simulink model "RADTRANS002"  (R2020b)
settings: Solver=VariableStepAuto  StartTime=0.0  StopTime=10.0  RelTol=1e-3
undefined symbols (not defined in the file): Line_110_C, Line_110_L, Line_110_R, Line_220_C, Line_220_L, Line_220_R, Line_35_C, Line_35_L, Line_35_R, Line_6_L, Line_6_R, Sys_f_Hz, Sys_V_net_kV, Tr_110_35_L_pu, Tr_110_35_R_pu, Tr_110_35_Sn_VA, Tr_110_35_V_HV_kV, Tr_110_35_V_LV_kV, Tr_110_6_L_pu, Tr_110_6_R_pu, Tr_110_6_Sn_VA, Tr_110_6_V_HV_kV, Tr_110_6_V_LV_kV, Tr_220_110_L_pu, Tr_220_110_R_pu, Tr_220_110_Sn_VA, Tr_220_110_V_HV_kV, Tr_220_110_V_LV_kV, Tr_35_04_L_pu, Tr_35_04_R_pu, Tr_35_04_Sn_VA, Tr_35_04_V_HV_kV, Tr_35_04_V_LV_kV, Tr_6_04_L_pu, Tr_6_04_R_pu, Tr_6_04_Sn_VA, Tr_6_04_V_HV_kV, Tr_6_04_V_LV_kV, Ts_powergui
libraries: dspstat3 x288, powerlib x202, powerlib_meascontrol x72
(part 6 of 7)

== system RADTRANS002/M_OUT_Город_4_4 ==
  Iptg_48 : Display
      settings: Format=bank
  PQptg_48 : Scope  NumInputPorts=2
  "Power0 (3ph, Instantaneous)" : powerlib_meascontrol/Measurements/Power (3ph, Instantaneous)
  Pptg_48 : Display
      settings: Format=bank
  Qptg_48 : Display
      settings: Format=bank
  RMS3 : dspstat3/RMS  run=off  directionMode=Each column  dimension=1  InputProcessing=Columns as channels (frame based)  reset_popup=None
  RMS4 : dspstat3/RMS  run=off  directionMode=Each column  dimension=1  InputProcessing=Columns as channels (frame based)  reset_popup=None
  RMS48 : dspstat3/RMS  run=off  directionMode=Each column  dimension=1  InputProcessing=Columns as channels (frame based)  reset_popup=None
  RMSpt_48 : dspstat3/RMS  run=off  directionMode=Each column  dimension=1  InputProcessing=Columns as channels (frame based)  reset_popup=None
  Real-Ima to Complex : RealImagToComplex
  S : Abs
  SSptg_48 : Scope
  Sptg_48 : Display
      settings: Format=bank
  Three-Phase V-I Measurementpt_48 : powerlib/Measurements/Three-Phase V-I Measurement  VoltageMeasurement=phase-to-ground  SetLabelV=off  LabelV=Vabc  Vpu=off  VpuLL=off  CurrentMeasurement=yes  SetLabelI=off  LabelI=Iabc  Ipu=off  Pbase=100e6  Vbase=500e3  OutputType=Complex  PhasorSimulation=off  PSBequivalent=0
  UIptg_48 : Scope  NumInputPorts=2
  Uptg_48 : Display
      settings: Format=bank
  a : PMIOPort  Side=Right
  b : PMIOPort  Port=2  Side=Right
  c : PMIOPort  Port=3  Side=Right
  A : PMIOPort  Port=4  Side=Left
  B : PMIOPort  Port=5  Side=Left
  C : PMIOPort  Port=6  Side=Left
  tag scope: I_ptg_48=global, P_ptg_48=global, Q_ptg_48=global, S_ptg_48=global, U_ptg_48=global
  wires:
  S/1 -> [S_ptg_48]
  Real-Ima to Complex/1 -> S/1
  [S_ptg_48] -> Sptg_48/1
  [S_ptg_48] -> SSptg_48/1
  [P_ptg_48] -> RMSpt_48/1
  RMSpt_48/1 -> Pptg_48/1
  RMS48/1 -> Qptg_48/1
  [U_ptg_48] -> RMS3/1
  RMS3/1 -> Uptg_48/1
  [P_ptg_48] -> Real-Ima to Complex/1
  [Q_ptg_48] -> RMS48/1
  [I_ptg_48] -> RMS4/1
  RMS4/1 -> Iptg_48/1
  [U_ptg_48] -> UIptg_48/1  "U"
  [P_ptg_48] -> PQptg_48/1  "P"
  [I_ptg_48] -> UIptg_48/2  "I"
  Three-Phase V-I Measurementpt_48/1 -> [U_ptg_48]
  [Q_ptg_48] -> Real-Ima to Complex/2
  Three-Phase V-I Measurementpt_48/2 -> [I_ptg_48]
  [U_ptg_48] -> "Power0 (3ph, Instantaneous)"/1
  [I_ptg_48] -> "Power0 (3ph, Instantaneous)"/2
  "Power0 (3ph, Instantaneous)"/2 -> [Q_ptg_48]
  "Power0 (3ph, Instantaneous)"/1 -> [P_ptg_48]
  [Q_ptg_48] -> PQptg_48/2  "Q"
  connections:
  Three-Phase V-I Measurementpt_48/LConn1 -- A/RConn1
  Three-Phase V-I Measurementpt_48/RConn1 -- a/RConn1
  Three-Phase V-I Measurementpt_48/LConn2 -- B/RConn1
  Three-Phase V-I Measurementpt_48/LConn3 -- C/RConn1
  Three-Phase V-I Measurementpt_48/RConn3 -- c/RConn1
  Three-Phase V-I Measurementpt_48/RConn2 -- b/RConn1

== system RADTRANS002/M_OUT_Город_5_1 ==
  Iptg_54 : Display
      settings: Format=bank
  PQptg_54 : Scope  NumInputPorts=2
  "Power0 (3ph, Instantaneous)" : powerlib_meascontrol/Measurements/Power (3ph, Instantaneous)
  Pptg_54 : Display
      settings: Format=bank
  Qptg_54 : Display
      settings: Format=bank
  RMS3 : dspstat3/RMS  run=off  directionMode=Each column  dimension=1  InputProcessing=Columns as channels (frame based)  reset_popup=None
  RMS4 : dspstat3/RMS  run=off  directionMode=Each column  dimension=1  InputProcessing=Columns as channels (frame based)  reset_popup=None
  RMS54 : dspstat3/RMS  run=off  directionMode=Each column  dimension=1  InputProcessing=Columns as channels (frame based)  reset_popup=None
  RMSpt_54 : dspstat3/RMS  run=off  directionMode=Each column  dimension=1  InputProcessing=Columns as channels (frame based)  reset_popup=None
  Real-Ima to Complex : RealImagToComplex
  S : Abs
  SSptg_54 : Scope
  Sptg_54 : Display
      settings: Format=bank
  Three-Phase V-I Measurementpt_54 : powerlib/Measurements/Three-Phase V-I Measurement  VoltageMeasurement=phase-to-ground  SetLabelV=off  LabelV=Vabc  Vpu=off  VpuLL=off  CurrentMeasurement=yes  SetLabelI=off  LabelI=Iabc  Ipu=off  Pbase=100e6  Vbase=500e3  OutputType=Complex  PhasorSimulation=off  PSBequivalent=0
  UIptg_54 : Scope  NumInputPorts=2
  Uptg_54 : Display
      settings: Format=bank
  a : PMIOPort  Side=Right
  b : PMIOPort  Port=2  Side=Right
  c : PMIOPort  Port=3  Side=Right
  A : PMIOPort  Port=4  Side=Left
  B : PMIOPort  Port=5  Side=Left
  C : PMIOPort  Port=6  Side=Left
  tag scope: I_ptg_54=global, P_ptg_54=global, Q_ptg_54=global, S_ptg_54=global, U_ptg_54=global
  wires:
  S/1 -> [S_ptg_54]
  Real-Ima to Complex/1 -> S/1
  [S_ptg_54] -> Sptg_54/1
  [S_ptg_54] -> SSptg_54/1
  [P_ptg_54] -> RMSpt_54/1
  RMSpt_54/1 -> Pptg_54/1
  RMS54/1 -> Qptg_54/1
  [U_ptg_54] -> RMS3/1
  RMS3/1 -> Uptg_54/1
  [P_ptg_54] -> Real-Ima to Complex/1
  [Q_ptg_54] -> RMS54/1
  [I_ptg_54] -> RMS4/1
  RMS4/1 -> Iptg_54/1
  [U_ptg_54] -> UIptg_54/1  "U"
  [P_ptg_54] -> PQptg_54/1  "P"
  [I_ptg_54] -> UIptg_54/2  "I"
  Three-Phase V-I Measurementpt_54/1 -> [U_ptg_54]
  [Q_ptg_54] -> Real-Ima to Complex/2
  Three-Phase V-I Measurementpt_54/2 -> [I_ptg_54]
  [U_ptg_54] -> "Power0 (3ph, Instantaneous)"/1
  [I_ptg_54] -> "Power0 (3ph, Instantaneous)"/2
  "Power0 (3ph, Instantaneous)"/2 -> [Q_ptg_54]
  "Power0 (3ph, Instantaneous)"/1 -> [P_ptg_54]
  [Q_ptg_54] -> PQptg_54/2  "Q"
  connections:
  Three-Phase V-I Measurementpt_54/LConn1 -- A/RConn1
  Three-Phase V-I Measurementpt_54/RConn1 -- a/RConn1
  Three-Phase V-I Measurementpt_54/LConn2 -- B/RConn1
  Three-Phase V-I Measurementpt_54/LConn3 -- C/RConn1
  Three-Phase V-I Measurementpt_54/RConn3 -- c/RConn1
  Three-Phase V-I Measurementpt_54/RConn2 -- b/RConn1

== system RADTRANS002/M_OUT_Город_5_2 ==
  Iptg_56 : Display
      settings: Format=bank
  PQptg_56 : Scope  NumInputPorts=2
  "Power0 (3ph, Instantaneous)" : powerlib_meascontrol/Measurements/Power (3ph, Instantaneous)
  Pptg_56 : Display
      settings: Format=bank
  Qptg_56 : Display
      settings: Format=bank
  RMS3 : dspstat3/RMS  run=off  directionMode=Each column  dimension=1  InputProcessing=Columns as channels (frame based)  reset_popup=None
  RMS4 : dspstat3/RMS  run=off  directionMode=Each column  dimension=1  InputProcessing=Columns as channels (frame based)  reset_popup=None
  RMS56 : dspstat3/RMS  run=off  directionMode=Each column  dimension=1  InputProcessing=Columns as channels (frame based)  reset_popup=None
  RMSpt_56 : dspstat3/RMS  run=off  directionMode=Each column  dimension=1  InputProcessing=Columns as channels (frame based)  reset_popup=None
  Real-Ima to Complex : RealImagToComplex
  S : Abs
  SSptg_56 : Scope
  Sptg_56 : Display
      settings: Format=bank
  Three-Phase V-I Measurementpt_56 : powerlib/Measurements/Three-Phase V-I Measurement  VoltageMeasurement=phase-to-ground  SetLabelV=off  LabelV=Vabc  Vpu=off  VpuLL=off  CurrentMeasurement=yes  SetLabelI=off  LabelI=Iabc  Ipu=off  Pbase=100e6  Vbase=500e3  OutputType=Complex  PhasorSimulation=off  PSBequivalent=0
  UIptg_56 : Scope  NumInputPorts=2
  Uptg_56 : Display
      settings: Format=bank
  a : PMIOPort  Side=Right
  b : PMIOPort  Port=2  Side=Right
  c : PMIOPort  Port=3  Side=Right
  A : PMIOPort  Port=4  Side=Left
  B : PMIOPort  Port=5  Side=Left
  C : PMIOPort  Port=6  Side=Left
  tag scope: I_ptg_56=global, P_ptg_56=global, Q_ptg_56=global, S_ptg_56=global, U_ptg_56=global
  wires:
  S/1 -> [S_ptg_56]
  Real-Ima to Complex/1 -> S/1
  [S_ptg_56] -> Sptg_56/1
  [S_ptg_56] -> SSptg_56/1
  [P_ptg_56] -> RMSpt_56/1
  RMSpt_56/1 -> Pptg_56/1
  RMS56/1 -> Qptg_56/1
  [U_ptg_56] -> RMS3/1
  RMS3/1 -> Uptg_56/1
  [P_ptg_56] -> Real-Ima to Complex/1
  [Q_ptg_56] -> RMS56/1
  [I_ptg_56] -> RMS4/1
  RMS4/1 -> Iptg_56/1
  [U_ptg_56] -> UIptg_56/1  "U"
  [P_ptg_56] -> PQptg_56/1  "P"
  [I_ptg_56] -> UIptg_56/2  "I"
  Three-Phase V-I Measurementpt_56/1 -> [U_ptg_56]
  [Q_ptg_56] -> Real-Ima to Complex/2
  Three-Phase V-I Measurementpt_56/2 -> [I_ptg_56]
  [U_ptg_56] -> "Power0 (3ph, Instantaneous)"/1
  [I_ptg_56] -> "Power0 (3ph, Instantaneous)"/2
  "Power0 (3ph, Instantaneous)"/2 -> [Q_ptg_56]
  "Power0 (3ph, Instantaneous)"/1 -> [P_ptg_56]
  [Q_ptg_56] -> PQptg_56/2  "Q"
  connections:
  Three-Phase V-I Measurementpt_56/LConn1 -- A/RConn1
  Three-Phase V-I Measurementpt_56/RConn1 -- a/RConn1
  Three-Phase V-I Measurementpt_56/LConn2 -- B/RConn1
  Three-Phase V-I Measurementpt_56/LConn3 -- C/RConn1
  Three-Phase V-I Measurementpt_56/RConn3 -- c/RConn1
  Three-Phase V-I Measurementpt_56/RConn2 -- b/RConn1

== system RADTRANS002/M_OUT_Город_5_3 ==
  Iptg_58 : Display
      settings: Format=bank
  PQptg_58 : Scope  NumInputPorts=2
  "Power0 (3ph, Instantaneous)" : powerlib_meascontrol/Measurements/Power (3ph, Instantaneous)
  Pptg_58 : Display
      settings: Format=bank
  Qptg_58 : Display
      settings: Format=bank
  RMS3 : dspstat3/RMS  run=off  directionMode=Each column  dimension=1  InputProcessing=Columns as channels (frame based)  reset_popup=None
  RMS4 : dspstat3/RMS  run=off  directionMode=Each column  dimension=1  InputProcessing=Columns as channels (frame based)  reset_popup=None
  RMS58 : dspstat3/RMS  run=off  directionMode=Each column  dimension=1  InputProcessing=Columns as channels (frame based)  reset_popup=None
  RMSpt_58 : dspstat3/RMS  run=off  directionMode=Each column  dimension=1  InputProcessing=Columns as channels (frame based)  reset_popup=None
  Real-Ima to Complex : RealImagToComplex
  S : Abs
  SSptg_58 : Scope
  Sptg_58 : Display
      settings: Format=bank
  Three-Phase V-I Measurementpt_58 : powerlib/Measurements/Three-Phase V-I Measurement  VoltageMeasurement=phase-to-ground  SetLabelV=off  LabelV=Vabc  Vpu=off  VpuLL=off  CurrentMeasurement=yes  SetLabelI=off  LabelI=Iabc  Ipu=off  Pbase=100e6  Vbase=500e3  OutputType=Complex  PhasorSimulation=off  PSBequivalent=0
  UIptg_58 : Scope  NumInputPorts=2
  Uptg_58 : Display
      settings: Format=bank
  a : PMIOPort  Side=Right
  b : PMIOPort  Port=2  Side=Right
  c : PMIOPort  Port=3  Side=Right
  A : PMIOPort  Port=4  Side=Left
  B : PMIOPort  Port=5  Side=Left
  C : PMIOPort  Port=6  Side=Left
  tag scope: I_ptg_58=global, P_ptg_58=global, Q_ptg_58=global, S_ptg_58=global, U_ptg_58=global
  wires:
  S/1 -> [S_ptg_58]
  Real-Ima to Complex/1 -> S/1
  [S_ptg_58] -> Sptg_58/1
  [S_ptg_58] -> SSptg_58/1
  [P_ptg_58] -> RMSpt_58/1
  RMSpt_58/1 -> Pptg_58/1
  RMS58/1 -> Qptg_58/1
  [U_ptg_58] -> RMS3/1
  RMS3/1 -> Uptg_58/1
  [P_ptg_58] -> Real-Ima to Complex/1
  [Q_ptg_58] -> RMS58/1
  [I_ptg_58] -> RMS4/1
  RMS4/1 -> Iptg_58/1
  [U_ptg_58] -> UIptg_58/1  "U"
  [P_ptg_58] -> PQptg_58/1  "P"
  [I_ptg_58] -> UIptg_58/2  "I"
  Three-Phase V-I Measurementpt_58/1 -> [U_ptg_58]
  [Q_ptg_58] -> Real-Ima to Complex/2
  Three-Phase V-I Measurementpt_58/2 -> [I_ptg_58]
  [U_ptg_58] -> "Power0 (3ph, Instantaneous)"/1
  [I_ptg_58] -> "Power0 (3ph, Instantaneous)"/2
  "Power0 (3ph, Instantaneous)"/2 -> [Q_ptg_58]
  "Power0 (3ph, Instantaneous)"/1 -> [P_ptg_58]
  [Q_ptg_58] -> PQptg_58/2  "Q"
  connections:
  Three-Phase V-I Measurementpt_58/LConn1 -- A/RConn1
  Three-Phase V-I Measurementpt_58/RConn1 -- a/RConn1
  Three-Phase V-I Measurementpt_58/LConn2 -- B/RConn1
  Three-Phase V-I Measurementpt_58/LConn3 -- C/RConn1
  Three-Phase V-I Measurementpt_58/RConn3 -- c/RConn1
  Three-Phase V-I Measurementpt_58/RConn2 -- b/RConn1

== system RADTRANS002/M_OUT_Город_5_4 ==
  Iptg_60 : Display
      settings: Format=bank
  PQptg_60 : Scope  NumInputPorts=2
  "Power0 (3ph, Instantaneous)" : powerlib_meascontrol/Measurements/Power (3ph, Instantaneous)
  Pptg_60 : Display
      settings: Format=bank
  Qptg_60 : Display
      settings: Format=bank
  RMS3 : dspstat3/RMS  run=off  directionMode=Each column  dimension=1  InputProcessing=Columns as channels (frame based)  reset_popup=None
  RMS4 : dspstat3/RMS  run=off  directionMode=Each column  dimension=1  InputProcessing=Columns as channels (frame based)  reset_popup=None
  RMS60 : dspstat3/RMS  run=off  directionMode=Each column  dimension=1  InputProcessing=Columns as channels (frame based)  reset_popup=None
  RMSpt_60 : dspstat3/RMS  run=off  directionMode=Each column  dimension=1  InputProcessing=Columns as channels (frame based)  reset_popup=None
  Real-Ima to Complex : RealImagToComplex
  S : Abs
  SSptg_60 : Scope
  Sptg_60 : Display
      settings: Format=bank
  Three-Phase V-I Measurementpt_60 : powerlib/Measurements/Three-Phase V-I Measurement  VoltageMeasurement=phase-to-ground  SetLabelV=off  LabelV=Vabc  Vpu=off  VpuLL=off  CurrentMeasurement=yes  SetLabelI=off  LabelI=Iabc  Ipu=off  Pbase=100e6  Vbase=500e3  OutputType=Complex  PhasorSimulation=off  PSBequivalent=0
  UIptg_60 : Scope  NumInputPorts=2
  Uptg_60 : Display
      settings: Format=bank
  a : PMIOPort  Side=Right
  b : PMIOPort  Port=2  Side=Right
  c : PMIOPort  Port=3  Side=Right
  A : PMIOPort  Port=4  Side=Left
  B : PMIOPort  Port=5  Side=Left
  C : PMIOPort  Port=6  Side=Left
  tag scope: I_ptg_60=global, P_ptg_60=global, Q_ptg_60=global, S_ptg_60=global, U_ptg_60=global
  wires:
  S/1 -> [S_ptg_60]
  Real-Ima to Complex/1 -> S/1
  [S_ptg_60] -> Sptg_60/1
  [S_ptg_60] -> SSptg_60/1
  [P_ptg_60] -> RMSpt_60/1
  RMSpt_60/1 -> Pptg_60/1
  RMS60/1 -> Qptg_60/1
  [U_ptg_60] -> RMS3/1
  RMS3/1 -> Uptg_60/1
  [P_ptg_60] -> Real-Ima to Complex/1
  [Q_ptg_60] -> RMS60/1
  [I_ptg_60] -> RMS4/1
  RMS4/1 -> Iptg_60/1
  [U_ptg_60] -> UIptg_60/1  "U"
  [P_ptg_60] -> PQptg_60/1  "P"
  [I_ptg_60] -> UIptg_60/2  "I"
  Three-Phase V-I Measurementpt_60/1 -> [U_ptg_60]
  [Q_ptg_60] -> Real-Ima to Complex/2
  Three-Phase V-I Measurementpt_60/2 -> [I_ptg_60]
  [U_ptg_60] -> "Power0 (3ph, Instantaneous)"/1
  [I_ptg_60] -> "Power0 (3ph, Instantaneous)"/2
  "Power0 (3ph, Instantaneous)"/2 -> [Q_ptg_60]
  "Power0 (3ph, Instantaneous)"/1 -> [P_ptg_60]
  [Q_ptg_60] -> PQptg_60/2  "Q"
  connections:
  Three-Phase V-I Measurementpt_60/LConn1 -- A/RConn1
  Three-Phase V-I Measurementpt_60/RConn1 -- a/RConn1
  Three-Phase V-I Measurementpt_60/LConn2 -- B/RConn1
  Three-Phase V-I Measurementpt_60/LConn3 -- C/RConn1
  Three-Phase V-I Measurementpt_60/RConn3 -- c/RConn1
  Three-Phase V-I Measurementpt_60/RConn2 -- b/RConn1

== system RADTRANS002/M_OUT_Город_6_1 ==
  Iptg_66 : Display
      settings: Format=bank
  PQptg_66 : Scope  NumInputPorts=2
  "Power0 (3ph, Instantaneous)" : powerlib_meascontrol/Measurements/Power (3ph, Instantaneous)
  Pptg_66 : Display
      settings: Format=bank
  Qptg_66 : Display
      settings: Format=bank
  RMS3 : dspstat3/RMS  run=off  directionMode=Each column  dimension=1  InputProcessing=Columns as channels (frame based)  reset_popup=None
  RMS4 : dspstat3/RMS  run=off  directionMode=Each column  dimension=1  InputProcessing=Columns as channels (frame based)  reset_popup=None
  RMS66 : dspstat3/RMS  run=off  directionMode=Each column  dimension=1  InputProcessing=Columns as channels (frame based)  reset_popup=None
  RMSpt_66 : dspstat3/RMS  run=off  directionMode=Each column  dimension=1  InputProcessing=Columns as channels (frame based)  reset_popup=None
  Real-Ima to Complex : RealImagToComplex
  S : Abs
  SSptg_66 : Scope
  Sptg_66 : Display
      settings: Format=bank
  Three-Phase V-I Measurementpt_66 : powerlib/Measurements/Three-Phase V-I Measurement  VoltageMeasurement=phase-to-ground  SetLabelV=off  LabelV=Vabc  Vpu=off  VpuLL=off  CurrentMeasurement=yes  SetLabelI=off  LabelI=Iabc  Ipu=off  Pbase=100e6  Vbase=500e3  OutputType=Complex  PhasorSimulation=off  PSBequivalent=0
  UIptg_66 : Scope  NumInputPorts=2
  Uptg_66 : Display
      settings: Format=bank
  a : PMIOPort  Side=Right
  b : PMIOPort  Port=2  Side=Right
  c : PMIOPort  Port=3  Side=Right
  A : PMIOPort  Port=4  Side=Left
  B : PMIOPort  Port=5  Side=Left
  C : PMIOPort  Port=6  Side=Left
  tag scope: I_ptg_66=global, P_ptg_66=global, Q_ptg_66=global, S_ptg_66=global, U_ptg_66=global
  wires:
  S/1 -> [S_ptg_66]
  Real-Ima to Complex/1 -> S/1
  [S_ptg_66] -> Sptg_66/1
  [S_ptg_66] -> SSptg_66/1
  [P_ptg_66] -> RMSpt_66/1
  RMSpt_66/1 -> Pptg_66/1
  RMS66/1 -> Qptg_66/1
  [U_ptg_66] -> RMS3/1
  RMS3/1 -> Uptg_66/1
  [P_ptg_66] -> Real-Ima to Complex/1
  [Q_ptg_66] -> RMS66/1
  [I_ptg_66] -> RMS4/1
  RMS4/1 -> Iptg_66/1
  [U_ptg_66] -> UIptg_66/1  "U"
  [P_ptg_66] -> PQptg_66/1  "P"
  [I_ptg_66] -> UIptg_66/2  "I"
  Three-Phase V-I Measurementpt_66/1 -> [U_ptg_66]
  [Q_ptg_66] -> Real-Ima to Complex/2
  Three-Phase V-I Measurementpt_66/2 -> [I_ptg_66]
  [U_ptg_66] -> "Power0 (3ph, Instantaneous)"/1
  [I_ptg_66] -> "Power0 (3ph, Instantaneous)"/2
  "Power0 (3ph, Instantaneous)"/2 -> [Q_ptg_66]
  "Power0 (3ph, Instantaneous)"/1 -> [P_ptg_66]
  [Q_ptg_66] -> PQptg_66/2  "Q"
  connections:
  Three-Phase V-I Measurementpt_66/LConn1 -- A/RConn1
  Three-Phase V-I Measurementpt_66/RConn1 -- a/RConn1
  Three-Phase V-I Measurementpt_66/LConn2 -- B/RConn1
  Three-Phase V-I Measurementpt_66/LConn3 -- C/RConn1
  Three-Phase V-I Measurementpt_66/RConn3 -- c/RConn1
  Three-Phase V-I Measurementpt_66/RConn2 -- b/RConn1

== system RADTRANS002/M_OUT_Город_6_2 ==
  Iptg_68 : Display
      settings: Format=bank
  PQptg_68 : Scope  NumInputPorts=2
  "Power0 (3ph, Instantaneous)" : powerlib_meascontrol/Measurements/Power (3ph, Instantaneous)
  Pptg_68 : Display
      settings: Format=bank
  Qptg_68 : Display
      settings: Format=bank
  RMS3 : dspstat3/RMS  run=off  directionMode=Each column  dimension=1  InputProcessing=Columns as channels (frame based)  reset_popup=None
  RMS4 : dspstat3/RMS  run=off  directionMode=Each column  dimension=1  InputProcessing=Columns as channels (frame based)  reset_popup=None
  RMS68 : dspstat3/RMS  run=off  directionMode=Each column  dimension=1  InputProcessing=Columns as channels (frame based)  reset_popup=None
  RMSpt_68 : dspstat3/RMS  run=off  directionMode=Each column  dimension=1  InputProcessing=Columns as channels (frame based)  reset_popup=None
  Real-Ima to Complex : RealImagToComplex
  S : Abs
  SSptg_68 : Scope
  Sptg_68 : Display
      settings: Format=bank
  Three-Phase V-I Measurementpt_68 : powerlib/Measurements/Three-Phase V-I Measurement  VoltageMeasurement=phase-to-ground  SetLabelV=off  LabelV=Vabc  Vpu=off  VpuLL=off  CurrentMeasurement=yes  SetLabelI=off  LabelI=Iabc  Ipu=off  Pbase=100e6  Vbase=500e3  OutputType=Complex  PhasorSimulation=off  PSBequivalent=0
  UIptg_68 : Scope  NumInputPorts=2
  Uptg_68 : Display
      settings: Format=bank
  a : PMIOPort  Side=Right
  b : PMIOPort  Port=2  Side=Right
  c : PMIOPort  Port=3  Side=Right
  A : PMIOPort  Port=4  Side=Left
  B : PMIOPort  Port=5  Side=Left
  C : PMIOPort  Port=6  Side=Left
  tag scope: I_ptg_68=global, P_ptg_68=global, Q_ptg_68=global, S_ptg_68=global, U_ptg_68=global
  wires:
  S/1 -> [S_ptg_68]
  Real-Ima to Complex/1 -> S/1
  [S_ptg_68] -> Sptg_68/1
  [S_ptg_68] -> SSptg_68/1
  [P_ptg_68] -> RMSpt_68/1
  RMSpt_68/1 -> Pptg_68/1
  RMS68/1 -> Qptg_68/1
  [U_ptg_68] -> RMS3/1
  RMS3/1 -> Uptg_68/1
  [P_ptg_68] -> Real-Ima to Complex/1
  [Q_ptg_68] -> RMS68/1
  [I_ptg_68] -> RMS4/1
  RMS4/1 -> Iptg_68/1
  [U_ptg_68] -> UIptg_68/1  "U"
  [P_ptg_68] -> PQptg_68/1  "P"
  [I_ptg_68] -> UIptg_68/2  "I"
  Three-Phase V-I Measurementpt_68/1 -> [U_ptg_68]
  [Q_ptg_68] -> Real-Ima to Complex/2
  Three-Phase V-I Measurementpt_68/2 -> [I_ptg_68]
  [U_ptg_68] -> "Power0 (3ph, Instantaneous)"/1
  [I_ptg_68] -> "Power0 (3ph, Instantaneous)"/2
  "Power0 (3ph, Instantaneous)"/2 -> [Q_ptg_68]
  "Power0 (3ph, Instantaneous)"/1 -> [P_ptg_68]
  [Q_ptg_68] -> PQptg_68/2  "Q"
  connections:
  Three-Phase V-I Measurementpt_68/LConn1 -- A/RConn1
  Three-Phase V-I Measurementpt_68/RConn1 -- a/RConn1
  Three-Phase V-I Measurementpt_68/LConn2 -- B/RConn1
  Three-Phase V-I Measurementpt_68/LConn3 -- C/RConn1
  Three-Phase V-I Measurementpt_68/RConn3 -- c/RConn1
  Three-Phase V-I Measurementpt_68/RConn2 -- b/RConn1

== system RADTRANS002/M_OUT_Город_6_3 ==
  Iptg_70 : Display
      settings: Format=bank
  PQptg_70 : Scope  NumInputPorts=2
  "Power0 (3ph, Instantaneous)" : powerlib_meascontrol/Measurements/Power (3ph, Instantaneous)
  Pptg_70 : Display
      settings: Format=bank
  Qptg_70 : Display
      settings: Format=bank
  RMS3 : dspstat3/RMS  run=off  directionMode=Each column  dimension=1  InputProcessing=Columns as channels (frame based)  reset_popup=None
  RMS4 : dspstat3/RMS  run=off  directionMode=Each column  dimension=1  InputProcessing=Columns as channels (frame based)  reset_popup=None
  RMS70 : dspstat3/RMS  run=off  directionMode=Each column  dimension=1  InputProcessing=Columns as channels (frame based)  reset_popup=None
  RMSpt_70 : dspstat3/RMS  run=off  directionMode=Each column  dimension=1  InputProcessing=Columns as channels (frame based)  reset_popup=None
  Real-Ima to Complex : RealImagToComplex
  S : Abs
  SSptg_70 : Scope
  Sptg_70 : Display
      settings: Format=bank
  Three-Phase V-I Measurementpt_70 : powerlib/Measurements/Three-Phase V-I Measurement  VoltageMeasurement=phase-to-ground  SetLabelV=off  LabelV=Vabc  Vpu=off  VpuLL=off  CurrentMeasurement=yes  SetLabelI=off  LabelI=Iabc  Ipu=off  Pbase=100e6  Vbase=500e3  OutputType=Complex  PhasorSimulation=off  PSBequivalent=0
  UIptg_70 : Scope  NumInputPorts=2
  Uptg_70 : Display
      settings: Format=bank
  a : PMIOPort  Side=Right
  b : PMIOPort  Port=2  Side=Right
  c : PMIOPort  Port=3  Side=Right
  A : PMIOPort  Port=4  Side=Left
  B : PMIOPort  Port=5  Side=Left
  C : PMIOPort  Port=6  Side=Left
  tag scope: I_ptg_70=global, P_ptg_70=global, Q_ptg_70=global, S_ptg_70=global, U_ptg_70=global
  wires:
  S/1 -> [S_ptg_70]
  Real-Ima to Complex/1 -> S/1
  [S_ptg_70] -> Sptg_70/1
  [S_ptg_70] -> SSptg_70/1
  [P_ptg_70] -> RMSpt_70/1
  RMSpt_70/1 -> Pptg_70/1
  RMS70/1 -> Qptg_70/1
  [U_ptg_70] -> RMS3/1
  RMS3/1 -> Uptg_70/1
  [P_ptg_70] -> Real-Ima to Complex/1
  [Q_ptg_70] -> RMS70/1
  [I_ptg_70] -> RMS4/1
  RMS4/1 -> Iptg_70/1
  [U_ptg_70] -> UIptg_70/1  "U"
  [P_ptg_70] -> PQptg_70/1  "P"
  [I_ptg_70] -> UIptg_70/2  "I"
  Three-Phase V-I Measurementpt_70/1 -> [U_ptg_70]
  [Q_ptg_70] -> Real-Ima to Complex/2
  Three-Phase V-I Measurementpt_70/2 -> [I_ptg_70]
  [U_ptg_70] -> "Power0 (3ph, Instantaneous)"/1
  [I_ptg_70] -> "Power0 (3ph, Instantaneous)"/2
  "Power0 (3ph, Instantaneous)"/2 -> [Q_ptg_70]
  "Power0 (3ph, Instantaneous)"/1 -> [P_ptg_70]
  [Q_ptg_70] -> PQptg_70/2  "Q"
  connections:
  Three-Phase V-I Measurementpt_70/LConn1 -- A/RConn1
  Three-Phase V-I Measurementpt_70/RConn1 -- a/RConn1
  Three-Phase V-I Measurementpt_70/LConn2 -- B/RConn1
  Three-Phase V-I Measurementpt_70/LConn3 -- C/RConn1
  Three-Phase V-I Measurementpt_70/RConn3 -- c/RConn1
  Three-Phase V-I Measurementpt_70/RConn2 -- b/RConn1

== system RADTRANS002/M_OUT_Город_6_4 ==
  Iptg_72 : Display
      settings: Format=bank
  PQptg_72 : Scope  NumInputPorts=2
  "Power0 (3ph, Instantaneous)" : powerlib_meascontrol/Measurements/Power (3ph, Instantaneous)
  Pptg_72 : Display
      settings: Format=bank
  Qptg_72 : Display
      settings: Format=bank
  RMS3 : dspstat3/RMS  run=off  directionMode=Each column  dimension=1  InputProcessing=Columns as channels (frame based)  reset_popup=None
  RMS4 : dspstat3/RMS  run=off  directionMode=Each column  dimension=1  InputProcessing=Columns as channels (frame based)  reset_popup=None
  RMS72 : dspstat3/RMS  run=off  directionMode=Each column  dimension=1  InputProcessing=Columns as channels (frame based)  reset_popup=None
  RMSpt_72 : dspstat3/RMS  run=off  directionMode=Each column  dimension=1  InputProcessing=Columns as channels (frame based)  reset_popup=None
  Real-Ima to Complex : RealImagToComplex
  S : Abs
  SSptg_72 : Scope
  Sptg_72 : Display
      settings: Format=bank
  Three-Phase V-I Measurementpt_72 : powerlib/Measurements/Three-Phase V-I Measurement  VoltageMeasurement=phase-to-ground  SetLabelV=off  LabelV=Vabc  Vpu=off  VpuLL=off  CurrentMeasurement=yes  SetLabelI=off  LabelI=Iabc  Ipu=off  Pbase=100e6  Vbase=500e3  OutputType=Complex  PhasorSimulation=off  PSBequivalent=0
  UIptg_72 : Scope  NumInputPorts=2
  Uptg_72 : Display
      settings: Format=bank
  a : PMIOPort  Side=Right
  b : PMIOPort  Port=2  Side=Right
  c : PMIOPort  Port=3  Side=Right
  A : PMIOPort  Port=4  Side=Left
  B : PMIOPort  Port=5  Side=Left
  C : PMIOPort  Port=6  Side=Left
  tag scope: I_ptg_72=global, P_ptg_72=global, Q_ptg_72=global, S_ptg_72=global, U_ptg_72=global
  wires:
  S/1 -> [S_ptg_72]
  Real-Ima to Complex/1 -> S/1
  [S_ptg_72] -> Sptg_72/1
  [S_ptg_72] -> SSptg_72/1
  [P_ptg_72] -> RMSpt_72/1
  RMSpt_72/1 -> Pptg_72/1
  RMS72/1 -> Qptg_72/1
  [U_ptg_72] -> RMS3/1
  RMS3/1 -> Uptg_72/1
  [P_ptg_72] -> Real-Ima to Complex/1
  [Q_ptg_72] -> RMS72/1
  [I_ptg_72] -> RMS4/1
  RMS4/1 -> Iptg_72/1
  [U_ptg_72] -> UIptg_72/1  "U"
  [P_ptg_72] -> PQptg_72/1  "P"
  [I_ptg_72] -> UIptg_72/2  "I"
  Three-Phase V-I Measurementpt_72/1 -> [U_ptg_72]
  [Q_ptg_72] -> Real-Ima to Complex/2
  Three-Phase V-I Measurementpt_72/2 -> [I_ptg_72]
  [U_ptg_72] -> "Power0 (3ph, Instantaneous)"/1
  [I_ptg_72] -> "Power0 (3ph, Instantaneous)"/2
  "Power0 (3ph, Instantaneous)"/2 -> [Q_ptg_72]
  "Power0 (3ph, Instantaneous)"/1 -> [P_ptg_72]
  [Q_ptg_72] -> PQptg_72/2  "Q"
  connections:
  Three-Phase V-I Measurementpt_72/LConn1 -- A/RConn1
  Three-Phase V-I Measurementpt_72/RConn1 -- a/RConn1
  Three-Phase V-I Measurementpt_72/LConn2 -- B/RConn1
  Three-Phase V-I Measurementpt_72/LConn3 -- C/RConn1
  Three-Phase V-I Measurementpt_72/RConn3 -- c/RConn1
  Three-Phase V-I Measurementpt_72/RConn2 -- b/RConn1

== system RADTRANS002/M_OUT_Завод_1_1 ==
  Iptg_2 : Display
      settings: Format=bank
  PQptg_2 : Scope  NumInputPorts=2
  "Power0 (3ph, Instantaneous)" : powerlib_meascontrol/Measurements/Power (3ph, Instantaneous)
  Pptg_2 : Display
      settings: Format=bank
  Qptg_2 : Display
      settings: Format=bank
  RMS2 : dspstat3/RMS  run=off  directionMode=Each column  dimension=1  InputProcessing=Columns as channels (frame based)  reset_popup=None
  RMS3 : dspstat3/RMS  run=off  directionMode=Each column  dimension=1  InputProcessing=Columns as channels (frame based)  reset_popup=None
  RMS4 : dspstat3/RMS  run=off  directionMode=Each column  dimension=1  InputProcessing=Columns as channels (frame based)  reset_popup=None
  RMSpt_2 : dspstat3/RMS  run=off  directionMode=Each column  dimension=1  InputProcessing=Columns as channels (frame based)  reset_popup=None
  Real-Ima to Complex : RealImagToComplex
  S : Abs
  SSptg_2 : Scope
  Sptg_2 : Display
      settings: Format=bank
  Three-Phase V-I Measurementpt_2 : powerlib/Measurements/Three-Phase V-I Measurement  VoltageMeasurement=phase-to-ground  SetLabelV=off  LabelV=Vabc  Vpu=off  VpuLL=off  CurrentMeasurement=yes  SetLabelI=off  LabelI=Iabc  Ipu=off  Pbase=100e6  Vbase=500e3  OutputType=Complex  PhasorSimulation=off  PSBequivalent=0
  UIptg_2 : Scope  NumInputPorts=2
  Uptg_2 : Display
      settings: Format=bank
  a : PMIOPort  Side=Right
  b : PMIOPort  Port=2  Side=Right
  c : PMIOPort  Port=3  Side=Right
  A : PMIOPort  Port=4  Side=Left
  B : PMIOPort  Port=5  Side=Left
  C : PMIOPort  Port=6  Side=Left
  tag scope: I_ptg_2=global, P_ptg_2=global, Q_ptg_2=global, S_ptg_2=global, U_ptg_2=global
  wires:
  S/1 -> [S_ptg_2]
  Real-Ima to Complex/1 -> S/1
  [S_ptg_2] -> Sptg_2/1
  [S_ptg_2] -> SSptg_2/1
  [P_ptg_2] -> RMSpt_2/1
  RMSpt_2/1 -> Pptg_2/1
  RMS2/1 -> Qptg_2/1
  [U_ptg_2] -> RMS3/1
  RMS3/1 -> Uptg_2/1
  [P_ptg_2] -> Real-Ima to Complex/1
  [Q_ptg_2] -> RMS2/1
  [I_ptg_2] -> RMS4/1
  RMS4/1 -> Iptg_2/1
  [U_ptg_2] -> UIptg_2/1  "U"
  [P_ptg_2] -> PQptg_2/1  "P"
  [I_ptg_2] -> UIptg_2/2  "I"
  Three-Phase V-I Measurementpt_2/1 -> [U_ptg_2]
  [Q_ptg_2] -> Real-Ima to Complex/2
  Three-Phase V-I Measurementpt_2/2 -> [I_ptg_2]
  [U_ptg_2] -> "Power0 (3ph, Instantaneous)"/1
  [I_ptg_2] -> "Power0 (3ph, Instantaneous)"/2
  "Power0 (3ph, Instantaneous)"/2 -> [Q_ptg_2]
  "Power0 (3ph, Instantaneous)"/1 -> [P_ptg_2]
  [Q_ptg_2] -> PQptg_2/2  "Q"
  connections:
  Three-Phase V-I Measurementpt_2/LConn1 -- A/RConn1
  Three-Phase V-I Measurementpt_2/RConn1 -- a/RConn1
  Three-Phase V-I Measurementpt_2/LConn2 -- B/RConn1
  Three-Phase V-I Measurementpt_2/LConn3 -- C/RConn1
  Three-Phase V-I Measurementpt_2/RConn3 -- c/RConn1
  Three-Phase V-I Measurementpt_2/RConn2 -- b/RConn1

== system RADTRANS002/M_OUT_Завод_1_2 ==
  Iptg_4 : Display
      settings: Format=bank
  PQptg_4 : Scope  NumInputPorts=2
  "Power0 (3ph, Instantaneous)" : powerlib_meascontrol/Measurements/Power (3ph, Instantaneous)
  Pptg_4 : Display
      settings: Format=bank
  Qptg_4 : Display
      settings: Format=bank
  RMS0 : dspstat3/RMS  run=off  directionMode=Each column  dimension=1  InputProcessing=Columns as channels (frame based)  reset_popup=None
  RMS3 : dspstat3/RMS  run=off  directionMode=Each column  dimension=1  InputProcessing=Columns as channels (frame based)  reset_popup=None
  RMS4 : dspstat3/RMS  run=off  directionMode=Each column  dimension=1  InputProcessing=Columns as channels (frame based)  reset_popup=None
  RMSpt_4 : dspstat3/RMS  run=off  directionMode=Each column  dimension=1  InputProcessing=Columns as channels (frame based)  reset_popup=None
  Real-Ima to Complex : RealImagToComplex
  S : Abs
  SSptg_4 : Scope
  Sptg_4 : Display
      settings: Format=bank
  Three-Phase V-I Measurementpt_4 : powerlib/Measurements/Three-Phase V-I Measurement  VoltageMeasurement=phase-to-ground  SetLabelV=off  LabelV=Vabc  Vpu=off  VpuLL=off  CurrentMeasurement=yes  SetLabelI=off  LabelI=Iabc  Ipu=off  Pbase=100e6  Vbase=500e3  OutputType=Complex  PhasorSimulation=off  PSBequivalent=0
  UIptg_4 : Scope  NumInputPorts=2
  Uptg_4 : Display
      settings: Format=bank
  a : PMIOPort  Side=Right
  b : PMIOPort  Port=2  Side=Right
  c : PMIOPort  Port=3  Side=Right
  A : PMIOPort  Port=4  Side=Left
  B : PMIOPort  Port=5  Side=Left
  C : PMIOPort  Port=6  Side=Left
  tag scope: I_ptg_4=global, P_ptg_4=global, Q_ptg_4=global, S_ptg_4=global, U_ptg_4=global
  wires:
  S/1 -> [S_ptg_4]
  Real-Ima to Complex/1 -> S/1
  [S_ptg_4] -> Sptg_4/1
  [S_ptg_4] -> SSptg_4/1
  [P_ptg_4] -> RMSpt_4/1
  RMSpt_4/1 -> Pptg_4/1
  RMS0/1 -> Qptg_4/1
  [U_ptg_4] -> RMS3/1
  RMS3/1 -> Uptg_4/1
  [P_ptg_4] -> Real-Ima to Complex/1
  [Q_ptg_4] -> RMS0/1
  [I_ptg_4] -> RMS4/1
  RMS4/1 -> Iptg_4/1
  [U_ptg_4] -> UIptg_4/1  "U"
  [P_ptg_4] -> PQptg_4/1  "P"
  [I_ptg_4] -> UIptg_4/2  "I"
  Three-Phase V-I Measurementpt_4/1 -> [U_ptg_4]
  [Q_ptg_4] -> Real-Ima to Complex/2
  Three-Phase V-I Measurementpt_4/2 -> [I_ptg_4]
  [U_ptg_4] -> "Power0 (3ph, Instantaneous)"/1
  [I_ptg_4] -> "Power0 (3ph, Instantaneous)"/2
  "Power0 (3ph, Instantaneous)"/2 -> [Q_ptg_4]
  "Power0 (3ph, Instantaneous)"/1 -> [P_ptg_4]
  [Q_ptg_4] -> PQptg_4/2  "Q"
  connections:
  Three-Phase V-I Measurementpt_4/LConn1 -- A/RConn1
  Three-Phase V-I Measurementpt_4/RConn1 -- a/RConn1
  Three-Phase V-I Measurementpt_4/LConn2 -- B/RConn1
  Three-Phase V-I Measurementpt_4/LConn3 -- C/RConn1
  Three-Phase V-I Measurementpt_4/RConn3 -- c/RConn1
  Three-Phase V-I Measurementpt_4/RConn2 -- b/RConn1

== system RADTRANS002/M_OUT_Завод_2_1 ==
  Iptg_14 : Display
      settings: Format=bank
  PQptg_14 : Scope  NumInputPorts=2
  "Power0 (3ph, Instantaneous)" : powerlib_meascontrol/Measurements/Power (3ph, Instantaneous)
  Pptg_14 : Display
      settings: Format=bank
  Qptg_14 : Display
      settings: Format=bank
  RMS14 : dspstat3/RMS  run=off  directionMode=Each column  dimension=1  InputProcessing=Columns as channels (frame based)  reset_popup=None
  RMS3 : dspstat3/RMS  run=off  directionMode=Each column  dimension=1  InputProcessing=Columns as channels (frame based)  reset_popup=None
  RMS4 : dspstat3/RMS  run=off  directionMode=Each column  dimension=1  InputProcessing=Columns as channels (frame based)  reset_popup=None
  RMSpt_14 : dspstat3/RMS  run=off  directionMode=Each column  dimension=1  InputProcessing=Columns as channels (frame based)  reset_popup=None
  Real-Ima to Complex : RealImagToComplex
  S : Abs
  SSptg_14 : Scope
  Sptg_14 : Display
      settings: Format=bank
  Three-Phase V-I Measurementpt_14 : powerlib/Measurements/Three-Phase V-I Measurement  VoltageMeasurement=phase-to-ground  SetLabelV=off  LabelV=Vabc  Vpu=off  VpuLL=off  CurrentMeasurement=yes  SetLabelI=off  LabelI=Iabc  Ipu=off  Pbase=100e6  Vbase=500e3  OutputType=Complex  PhasorSimulation=off  PSBequivalent=0
  UIptg_14 : Scope  NumInputPorts=2
  Uptg_14 : Display
      settings: Format=bank
  a : PMIOPort  Side=Right
  b : PMIOPort  Port=2  Side=Right
  c : PMIOPort  Port=3  Side=Right
  A : PMIOPort  Port=4  Side=Left
  B : PMIOPort  Port=5  Side=Left
  C : PMIOPort  Port=6  Side=Left
  tag scope: I_ptg_14=global, P_ptg_14=global, Q_ptg_14=global, S_ptg_14=global, U_ptg_14=global
  wires:
  S/1 -> [S_ptg_14]
  Real-Ima to Complex/1 -> S/1
  [S_ptg_14] -> Sptg_14/1
  [S_ptg_14] -> SSptg_14/1
  [P_ptg_14] -> RMSpt_14/1
  RMSpt_14/1 -> Pptg_14/1
  RMS14/1 -> Qptg_14/1
  [U_ptg_14] -> RMS3/1
  RMS3/1 -> Uptg_14/1
  [P_ptg_14] -> Real-Ima to Complex/1
  [Q_ptg_14] -> RMS14/1
  [I_ptg_14] -> RMS4/1
  RMS4/1 -> Iptg_14/1
  [U_ptg_14] -> UIptg_14/1  "U"
  [P_ptg_14] -> PQptg_14/1  "P"
  [I_ptg_14] -> UIptg_14/2  "I"
  Three-Phase V-I Measurementpt_14/1 -> [U_ptg_14]
  [Q_ptg_14] -> Real-Ima to Complex/2
  Three-Phase V-I Measurementpt_14/2 -> [I_ptg_14]
  [U_ptg_14] -> "Power0 (3ph, Instantaneous)"/1
  [I_ptg_14] -> "Power0 (3ph, Instantaneous)"/2
  "Power0 (3ph, Instantaneous)"/2 -> [Q_ptg_14]
  "Power0 (3ph, Instantaneous)"/1 -> [P_ptg_14]
  [Q_ptg_14] -> PQptg_14/2  "Q"
  connections:
  Three-Phase V-I Measurementpt_14/LConn1 -- A/RConn1
  Three-Phase V-I Measurementpt_14/RConn1 -- a/RConn1
  Three-Phase V-I Measurementpt_14/LConn2 -- B/RConn1
  Three-Phase V-I Measurementpt_14/LConn3 -- C/RConn1
  Three-Phase V-I Measurementpt_14/RConn3 -- c/RConn1
  Three-Phase V-I Measurementpt_14/RConn2 -- b/RConn1

== system RADTRANS002/M_OUT_Завод_2_2 ==
  Iptg_16 : Display
      settings: Format=bank
  PQptg_16 : Scope  NumInputPorts=2
  "Power0 (3ph, Instantaneous)" : powerlib_meascontrol/Measurements/Power (3ph, Instantaneous)
  Pptg_16 : Display
      settings: Format=bank
  Qptg_16 : Display
      settings: Format=bank
  RMS16 : dspstat3/RMS  run=off  directionMode=Each column  dimension=1  InputProcessing=Columns as channels (frame based)  reset_popup=None
  RMS3 : dspstat3/RMS  run=off  directionMode=Each column  dimension=1  InputProcessing=Columns as channels (frame based)  reset_popup=None
  RMS4 : dspstat3/RMS  run=off  directionMode=Each column  dimension=1  InputProcessing=Columns as channels (frame based)  reset_popup=None
  RMSpt_16 : dspstat3/RMS  run=off  directionMode=Each column  dimension=1  InputProcessing=Columns as channels (frame based)  reset_popup=None
  Real-Ima to Complex : RealImagToComplex
  S : Abs
  SSptg_16 : Scope
  Sptg_16 : Display
      settings: Format=bank
  Three-Phase V-I Measurementpt_16 : powerlib/Measurements/Three-Phase V-I Measurement  VoltageMeasurement=phase-to-ground  SetLabelV=off  LabelV=Vabc  Vpu=off  VpuLL=off  CurrentMeasurement=yes  SetLabelI=off  LabelI=Iabc  Ipu=off  Pbase=100e6  Vbase=500e3  OutputType=Complex  PhasorSimulation=off  PSBequivalent=0
  UIptg_16 : Scope  NumInputPorts=2
  Uptg_16 : Display
      settings: Format=bank
  a : PMIOPort  Side=Right
  b : PMIOPort  Port=2  Side=Right
  c : PMIOPort  Port=3  Side=Right
  A : PMIOPort  Port=4  Side=Left
  B : PMIOPort  Port=5  Side=Left
  C : PMIOPort  Port=6  Side=Left
  tag scope: I_ptg_16=global, P_ptg_16=global, Q_ptg_16=global, S_ptg_16=global, U_ptg_16=global
  wires:
  S/1 -> [S_ptg_16]
  Real-Ima to Complex/1 -> S/1
  [S_ptg_16] -> Sptg_16/1
  [S_ptg_16] -> SSptg_16/1
  [P_ptg_16] -> RMSpt_16/1
  RMSpt_16/1 -> Pptg_16/1
  RMS16/1 -> Qptg_16/1
  [U_ptg_16] -> RMS3/1
  RMS3/1 -> Uptg_16/1
  [P_ptg_16] -> Real-Ima to Complex/1
  [Q_ptg_16] -> RMS16/1
  [I_ptg_16] -> RMS4/1
  RMS4/1 -> Iptg_16/1
  [U_ptg_16] -> UIptg_16/1  "U"
  [P_ptg_16] -> PQptg_16/1  "P"
  [I_ptg_16] -> UIptg_16/2  "I"
  Three-Phase V-I Measurementpt_16/1 -> [U_ptg_16]
  [Q_ptg_16] -> Real-Ima to Complex/2
  Three-Phase V-I Measurementpt_16/2 -> [I_ptg_16]
  [U_ptg_16] -> "Power0 (3ph, Instantaneous)"/1
  [I_ptg_16] -> "Power0 (3ph, Instantaneous)"/2
  "Power0 (3ph, Instantaneous)"/2 -> [Q_ptg_16]
  "Power0 (3ph, Instantaneous)"/1 -> [P_ptg_16]
  [Q_ptg_16] -> PQptg_16/2  "Q"
  connections:
  Three-Phase V-I Measurementpt_16/LConn1 -- A/RConn1
  Three-Phase V-I Measurementpt_16/RConn1 -- a/RConn1
  Three-Phase V-I Measurementpt_16/LConn2 -- B/RConn1
  Three-Phase V-I Measurementpt_16/LConn3 -- C/RConn1
  Three-Phase V-I Measurementpt_16/RConn3 -- c/RConn1
  Three-Phase V-I Measurementpt_16/RConn2 -- b/RConn1

== system RADTRANS002/M_OUT_Завод_3_1 ==
  Iptg_26 : Display
      settings: Format=bank
  PQptg_26 : Scope  NumInputPorts=2
  "Power0 (3ph, Instantaneous)" : powerlib_meascontrol/Measurements/Power (3ph, Instantaneous)
  Pptg_26 : Display
      settings: Format=bank
  Qptg_26 : Display
      settings: Format=bank
  RMS26 : dspstat3/RMS  run=off  directionMode=Each column  dimension=1  InputProcessing=Columns as channels (frame based)  reset_popup=None
  RMS3 : dspstat3/RMS  run=off  directionMode=Each column  dimension=1  InputProcessing=Columns as channels (frame based)  reset_popup=None
  RMS4 : dspstat3/RMS  run=off  directionMode=Each column  dimension=1  InputProcessing=Columns as channels (frame based)  reset_popup=None
  RMSpt_26 : dspstat3/RMS  run=off  directionMode=Each column  dimension=1  InputProcessing=Columns as channels (frame based)  reset_popup=None
  Real-Ima to Complex : RealImagToComplex
  S : Abs
  SSptg_26 : Scope
  Sptg_26 : Display
      settings: Format=bank
  Three-Phase V-I Measurementpt_26 : powerlib/Measurements/Three-Phase V-I Measurement  VoltageMeasurement=phase-to-ground  SetLabelV=off  LabelV=Vabc  Vpu=off  VpuLL=off  CurrentMeasurement=yes  SetLabelI=off  LabelI=Iabc  Ipu=off  Pbase=100e6  Vbase=500e3  OutputType=Complex  PhasorSimulation=off  PSBequivalent=0
  UIptg_26 : Scope  NumInputPorts=2
  Uptg_26 : Display
      settings: Format=bank
  a : PMIOPort  Side=Right
  b : PMIOPort  Port=2  Side=Right
  c : PMIOPort  Port=3  Side=Right
  A : PMIOPort  Port=4  Side=Left
  B : PMIOPort  Port=5  Side=Left
  C : PMIOPort  Port=6  Side=Left
  tag scope: I_ptg_26=global, P_ptg_26=global, Q_ptg_26=global, S_ptg_26=global, U_ptg_26=global
  wires:
  S/1 -> [S_ptg_26]
  Real-Ima to Complex/1 -> S/1
  [S_ptg_26] -> Sptg_26/1
  [S_ptg_26] -> SSptg_26/1
  [P_ptg_26] -> RMSpt_26/1
  RMSpt_26/1 -> Pptg_26/1
  RMS26/1 -> Qptg_26/1
  [U_ptg_26] -> RMS3/1
  RMS3/1 -> Uptg_26/1
  [P_ptg_26] -> Real-Ima to Complex/1
  [Q_ptg_26] -> RMS26/1
  [I_ptg_26] -> RMS4/1
  RMS4/1 -> Iptg_26/1
  [U_ptg_26] -> UIptg_26/1  "U"
  [P_ptg_26] -> PQptg_26/1  "P"
  [I_ptg_26] -> UIptg_26/2  "I"
  Three-Phase V-I Measurementpt_26/1 -> [U_ptg_26]
  [Q_ptg_26] -> Real-Ima to Complex/2
  Three-Phase V-I Measurementpt_26/2 -> [I_ptg_26]
  [U_ptg_26] -> "Power0 (3ph, Instantaneous)"/1
  [I_ptg_26] -> "Power0 (3ph, Instantaneous)"/2
  "Power0 (3ph, Instantaneous)"/2 -> [Q_ptg_26]
  "Power0 (3ph, Instantaneous)"/1 -> [P_ptg_26]
  [Q_ptg_26] -> PQptg_26/2  "Q"
  connections:
  Three-Phase V-I Measurementpt_26/LConn1 -- A/RConn1
  Three-Phase V-I Measurementpt_26/RConn1 -- a/RConn1
  Three-Phase V-I Measurementpt_26/LConn2 -- B/RConn1
  Three-Phase V-I Measurementpt_26/LConn3 -- C/RConn1
  Three-Phase V-I Measurementpt_26/RConn3 -- c/RConn1
  Three-Phase V-I Measurementpt_26/RConn2 -- b/RConn1

== system RADTRANS002/M_OUT_Завод_3_2 ==
  Iptg_28 : Display
      settings: Format=bank
  PQptg_28 : Scope  NumInputPorts=2
  "Power0 (3ph, Instantaneous)" : powerlib_meascontrol/Measurements/Power (3ph, Instantaneous)
  Pptg_28 : Display
      settings: Format=bank
  Qptg_28 : Display
      settings: Format=bank
  RMS28 : dspstat3/RMS  run=off  directionMode=Each column  dimension=1  InputProcessing=Columns as channels (frame based)  reset_popup=None
  RMS3 : dspstat3/RMS  run=off  directionMode=Each column  dimension=1  InputProcessing=Columns as channels (frame based)  reset_popup=None
  RMS4 : dspstat3/RMS  run=off  directionMode=Each column  dimension=1  InputProcessing=Columns as channels (frame based)  reset_popup=None
  RMSpt_28 : dspstat3/RMS  run=off  directionMode=Each column  dimension=1  InputProcessing=Columns as channels (frame based)  reset_popup=None
  Real-Ima to Complex : RealImagToComplex
  S : Abs
  SSptg_28 : Scope
  Sptg_28 : Display
      settings: Format=bank
  Three-Phase V-I Measurementpt_28 : powerlib/Measurements/Three-Phase V-I Measurement  VoltageMeasurement=phase-to-ground  SetLabelV=off  LabelV=Vabc  Vpu=off  VpuLL=off  CurrentMeasurement=yes  SetLabelI=off  LabelI=Iabc  Ipu=off  Pbase=100e6  Vbase=500e3  OutputType=Complex  PhasorSimulation=off  PSBequivalent=0
  UIptg_28 : Scope  NumInputPorts=2
  Uptg_28 : Display
      settings: Format=bank
  a : PMIOPort  Side=Right
  b : PMIOPort  Port=2  Side=Right
  c : PMIOPort  Port=3  Side=Right
  A : PMIOPort  Port=4  Side=Left
  B : PMIOPort  Port=5  Side=Left
  C : PMIOPort  Port=6  Side=Left
  tag scope: I_ptg_28=global, P_ptg_28=global, Q_ptg_28=global, S_ptg_28=global, U_ptg_28=global
  wires:
  S/1 -> [S_ptg_28]
  Real-Ima to Complex/1 -> S/1
  [S_ptg_28] -> Sptg_28/1
  [S_ptg_28] -> SSptg_28/1
  [P_ptg_28] -> RMSpt_28/1
  RMSpt_28/1 -> Pptg_28/1
  RMS28/1 -> Qptg_28/1
  [U_ptg_28] -> RMS3/1
  RMS3/1 -> Uptg_28/1
  [P_ptg_28] -> Real-Ima to Complex/1
  [Q_ptg_28] -> RMS28/1
  [I_ptg_28] -> RMS4/1
  RMS4/1 -> Iptg_28/1
  [U_ptg_28] -> UIptg_28/1  "U"
  [P_ptg_28] -> PQptg_28/1  "P"
  [I_ptg_28] -> UIptg_28/2  "I"
  Three-Phase V-I Measurementpt_28/1 -> [U_ptg_28]
  [Q_ptg_28] -> Real-Ima to Complex/2
  Three-Phase V-I Measurementpt_28/2 -> [I_ptg_28]
  [U_ptg_28] -> "Power0 (3ph, Instantaneous)"/1
  [I_ptg_28] -> "Power0 (3ph, Instantaneous)"/2
  "Power0 (3ph, Instantaneous)"/2 -> [Q_ptg_28]
  "Power0 (3ph, Instantaneous)"/1 -> [P_ptg_28]
  [Q_ptg_28] -> PQptg_28/2  "Q"
  connections:
  Three-Phase V-I Measurementpt_28/LConn1 -- A/RConn1
  Three-Phase V-I Measurementpt_28/RConn1 -- a/RConn1
  Three-Phase V-I Measurementpt_28/LConn2 -- B/RConn1
  Three-Phase V-I Measurementpt_28/LConn3 -- C/RConn1
  Three-Phase V-I Measurementpt_28/RConn3 -- c/RConn1
  Three-Phase V-I Measurementpt_28/RConn2 -- b/RConn1

== system RADTRANS002/M_OUT_Завод_4_1 ==
  Iptg_38 : Display
      settings: Format=bank
  PQptg_38 : Scope  NumInputPorts=2
  "Power0 (3ph, Instantaneous)" : powerlib_meascontrol/Measurements/Power (3ph, Instantaneous)
  Pptg_38 : Display
      settings: Format=bank
  Qptg_38 : Display
      settings: Format=bank
  RMS3 : dspstat3/RMS  run=off  directionMode=Each column  dimension=1  InputProcessing=Columns as channels (frame based)  reset_popup=None
  RMS38 : dspstat3/RMS  run=off  directionMode=Each column  dimension=1  InputProcessing=Columns as channels (frame based)  reset_popup=None
  RMS4 : dspstat3/RMS  run=off  directionMode=Each column  dimension=1  InputProcessing=Columns as channels (frame based)  reset_popup=None
  RMSpt_38 : dspstat3/RMS  run=off  directionMode=Each column  dimension=1  InputProcessing=Columns as channels (frame based)  reset_popup=None
  Real-Ima to Complex : RealImagToComplex
  S : Abs
  SSptg_38 : Scope
  Sptg_38 : Display
      settings: Format=bank
  Three-Phase V-I Measurementpt_38 : powerlib/Measurements/Three-Phase V-I Measurement  VoltageMeasurement=phase-to-ground  SetLabelV=off  LabelV=Vabc  Vpu=off  VpuLL=off  CurrentMeasurement=yes  SetLabelI=off  LabelI=Iabc  Ipu=off  Pbase=100e6  Vbase=500e3  OutputType=Complex  PhasorSimulation=off  PSBequivalent=0
  UIptg_38 : Scope  NumInputPorts=2
  Uptg_38 : Display
      settings: Format=bank
  a : PMIOPort  Side=Right
  b : PMIOPort  Port=2  Side=Right
  c : PMIOPort  Port=3  Side=Right
  A : PMIOPort  Port=4  Side=Left
  B : PMIOPort  Port=5  Side=Left
  C : PMIOPort  Port=6  Side=Left
  tag scope: I_ptg_38=global, P_ptg_38=global, Q_ptg_38=global, S_ptg_38=global, U_ptg_38=global
  wires:
  S/1 -> [S_ptg_38]
  Real-Ima to Complex/1 -> S/1
  [S_ptg_38] -> Sptg_38/1
  [S_ptg_38] -> SSptg_38/1
  [P_ptg_38] -> RMSpt_38/1
  RMSpt_38/1 -> Pptg_38/1
  RMS38/1 -> Qptg_38/1
  [U_ptg_38] -> RMS3/1
  RMS3/1 -> Uptg_38/1
  [P_ptg_38] -> Real-Ima to Complex/1
  [Q_ptg_38] -> RMS38/1
  [I_ptg_38] -> RMS4/1
  RMS4/1 -> Iptg_38/1
  [U_ptg_38] -> UIptg_38/1  "U"
  [P_ptg_38] -> PQptg_38/1  "P"
  [I_ptg_38] -> UIptg_38/2  "I"
  Three-Phase V-I Measurementpt_38/1 -> [U_ptg_38]
  [Q_ptg_38] -> Real-Ima to Complex/2
  Three-Phase V-I Measurementpt_38/2 -> [I_ptg_38]
  [U_ptg_38] -> "Power0 (3ph, Instantaneous)"/1
  [I_ptg_38] -> "Power0 (3ph, Instantaneous)"/2
  "Power0 (3ph, Instantaneous)"/2 -> [Q_ptg_38]
  "Power0 (3ph, Instantaneous)"/1 -> [P_ptg_38]
  [Q_ptg_38] -> PQptg_38/2  "Q"
  connections:
  Three-Phase V-I Measurementpt_38/LConn1 -- A/RConn1
  Three-Phase V-I Measurementpt_38/RConn1 -- a/RConn1
  Three-Phase V-I Measurementpt_38/LConn2 -- B/RConn1
  Three-Phase V-I Measurementpt_38/LConn3 -- C/RConn1
  Three-Phase V-I Measurementpt_38/RConn3 -- c/RConn1
  Three-Phase V-I Measurementpt_38/RConn2 -- b/RConn1

== system RADTRANS002/M_OUT_Завод_4_2 ==
  Iptg_40 : Display
      settings: Format=bank
  PQptg_40 : Scope  NumInputPorts=2
  "Power0 (3ph, Instantaneous)" : powerlib_meascontrol/Measurements/Power (3ph, Instantaneous)
  Pptg_40 : Display
      settings: Format=bank
  Qptg_40 : Display
      settings: Format=bank
  RMS3 : dspstat3/RMS  run=off  directionMode=Each column  dimension=1  InputProcessing=Columns as channels (frame based)  reset_popup=None
  RMS4 : dspstat3/RMS  run=off  directionMode=Each column  dimension=1  InputProcessing=Columns as channels (frame based)  reset_popup=None
  RMS40 : dspstat3/RMS  run=off  directionMode=Each column  dimension=1  InputProcessing=Columns as channels (frame based)  reset_popup=None
  RMSpt_40 : dspstat3/RMS  run=off  directionMode=Each column  dimension=1  InputProcessing=Columns as channels (frame based)  reset_popup=None
  Real-Ima to Complex : RealImagToComplex
  S : Abs
  SSptg_40 : Scope
  Sptg_40 : Display
      settings: Format=bank
  Three-Phase V-I Measurementpt_40 : powerlib/Measurements/Three-Phase V-I Measurement  VoltageMeasurement=phase-to-ground  SetLabelV=off  LabelV=Vabc  Vpu=off  VpuLL=off  CurrentMeasurement=yes  SetLabelI=off  LabelI=Iabc  Ipu=off  Pbase=100e6  Vbase=500e3  OutputType=Complex  PhasorSimulation=off  PSBequivalent=0
  UIptg_40 : Scope  NumInputPorts=2
  Uptg_40 : Display
      settings: Format=bank
  a : PMIOPort  Side=Right
  b : PMIOPort  Port=2  Side=Right
  c : PMIOPort  Port=3  Side=Right
  A : PMIOPort  Port=4  Side=Left
  B : PMIOPort  Port=5  Side=Left
  C : PMIOPort  Port=6  Side=Left
  tag scope: I_ptg_40=global, P_ptg_40=global, Q_ptg_40=global, S_ptg_40=global, U_ptg_40=global
  wires:
  S/1 -> [S_ptg_40]
  Real-Ima to Complex/1 -> S/1
  [S_ptg_40] -> Sptg_40/1
  [S_ptg_40] -> SSptg_40/1
  [P_ptg_40] -> RMSpt_40/1
  RMSpt_40/1 -> Pptg_40/1
  RMS40/1 -> Qptg_40/1
  [U_ptg_40] -> RMS3/1
  RMS3/1 -> Uptg_40/1
  [P_ptg_40] -> Real-Ima to Complex/1
  [Q_ptg_40] -> RMS40/1
  [I_ptg_40] -> RMS4/1
  RMS4/1 -> Iptg_40/1
  [U_ptg_40] -> UIptg_40/1  "U"
  [P_ptg_40] -> PQptg_40/1  "P"
  [I_ptg_40] -> UIptg_40/2  "I"
  Three-Phase V-I Measurementpt_40/1 -> [U_ptg_40]
  [Q_ptg_40] -> Real-Ima to Complex/2
  Three-Phase V-I Measurementpt_40/2 -> [I_ptg_40]
  [U_ptg_40] -> "Power0 (3ph, Instantaneous)"/1
  [I_ptg_40] -> "Power0 (3ph, Instantaneous)"/2
  "Power0 (3ph, Instantaneous)"/2 -> [Q_ptg_40]
  "Power0 (3ph, Instantaneous)"/1 -> [P_ptg_40]
  [Q_ptg_40] -> PQptg_40/2  "Q"
  connections:
  Three-Phase V-I Measurementpt_40/LConn1 -- A/RConn1
  Three-Phase V-I Measurementpt_40/RConn1 -- a/RConn1
  Three-Phase V-I Measurementpt_40/LConn2 -- B/RConn1
  Three-Phase V-I Measurementpt_40/LConn3 -- C/RConn1
  Three-Phase V-I Measurementpt_40/RConn3 -- c/RConn1
  Three-Phase V-I Measurementpt_40/RConn2 -- b/RConn1
